simulink model "sistemaMotorCC_PID"  (R2018a)
settings: Solver=FixedStepAuto  StartTime=0.0  StopTime=119.98  RelTol=1e-3
PreLoadFcn:
  | % Motor Parameters
  | 
  | J=0.01;     %kg*m^2
  | b=0.1;      %N*m/(rad/s)
  | K=0.01;     %V/(rad/s)
  | R=1;        %Ohm
  | L=0.5;      %H
libraries: simulink x1
settings Model: Creator=deastman  LastModifiedBy=artur
settings DataIOCC: LimitDataPoints=on  SaveFormat=Array
settings OptimizationCC: ExpressionDepthLimit=2147483647  InitFltsAndDblsToZero=on  LifeSpan=inf
settings DebuggingCC: UnderspecifiedInitializationDetection=Classic  MergeDetectMultiDrivingBlocksExec=none  SolverPrmCheckMsg=warning  FcnCallInpInsideContextMsg=warning  StateNameClashWarn=warning  SFUnexpectedBacktrackingDiag=warning  SFNoUnconditionalDefaultTransitionDiag=warning  SFExecutionAtInitializationDiag=none
settings HardwareCC: ProdBitPerPointer=32  ProdBitPerSizeT=32  ProdBitPerPtrDiffT=32  ProdLargestAtomicFloat=None  ProdIntDivRoundTo=Undefined  ProdEndianess=Unspecified  ProdWordSize=32  ProdHWDeviceType=32-bit Generic
settings ModelReferenceCC: PropagateSignalLabelsOutOfModel=off
settings CodeAppCC: StateflowObjectComments=on
settings GRTTargetCC: TargetLangStandard=C89/C90 (ANSI)  GeneratePreprocessorConditionals=Disable all  CombineOutputUpdateFcns=off  GRTInterface=on
settings ConfigComp: CovMetricSettings=dw  CovHtmlReporting=on  CovSaveCumulativeToWorkspaceVar=on  CovSaveSingleToWorkspaceVar=on  CovExternalEMLEnable=off

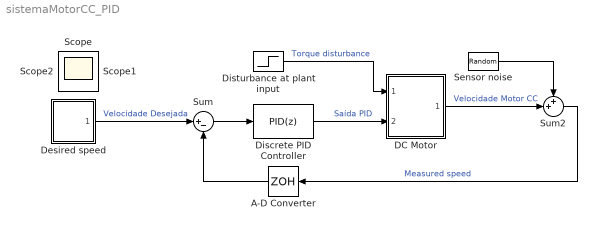
== system sistemaMotorCC_PID ==
  " Disturbance at plant input" : Step  Time=0  After=0  SampleTime=0
  A-D Converter : ZeroOrderHold  SampleTime=0.02
  DC Motor : Subsystem  mask(DC Motor){b=b, J=J, K=K, R=R, L=L}
      mask prompts: b "Damping:"; J "Inertia:"; K "Back EMF:"; R "Resistance:"; L "Inductance:"
      mask help: An ideal model of a DC Motor
      mask Help: This is <b>more elaborate<b> help.
      mask Display: image(imread('dcmotor.jpg'))
  Desired speed : Subsystem
  Discrete PID Controller : simulink/Continuous/PID Controller  Controller=PID  TimeDomain=Discrete-time  SampleTime=0.02  IntegratorMethod=Forward Euler  FilterMethod=Forward Euler  Form=Parallel  UseFilter=on  ControllerParametersSource=internal  P=5.6086  I=17.255  D=0  N=100  InitialConditionSource=internal  InitialConditionForIntegrator=0  InitialConditionForFilter=0  ExternalReset=none  LimitOutput=off  UpperSaturationLimit=10  LowerSaturationLimit=-10  LinearizeAsGain=on  AntiWindupMode=back-calculation  Kb=1  TrackingMode=off  Kt=1  PParamMin=[]  PParamMax=[]  IParamMin=[]  IParamMax=[]  DParamMin=[]  DParamMax=[]  NParamMin=[]  NParamMax=[]  KbParamMin=[]  KbParamMax=[]  KtParamMin=[]  KtParamMax=[]  POutMin=[]  POutMax=[]  IOutMin=[]  IOutMax=[]  DOutMin=[]  DOutMax=[]  NOutMin=[]  NOutMax=[]  KbOutMin=[]  KbOutMax=[]  KtOutMin=[]  KtOutMax=[]  IntegratorOutMin=[]  IntegratorOutMax=[]  FilterOutMin=[]  FilterOutMax=[]  SumOutMin=[]  SumOutMax=[]  SumI1OutMin=[]  SumI1OutMax=[]  SumI2OutMin=[]  SumI2OutMax=[]  SumI3OutMin=[]  SumI3OutMax=[]  SumDOutMin=[]  SumDOutMax=[]  SaturationOutMin=[]  SaturationOutMax=[]  IntegratorContinuousStateAttributes=''  IntegratorStateMustResolveToSignalObject=off  IntegratorRTWStateStorageClass=Auto  FilterContinuousStateAttributes=''  FilterStateMustResolveToSignalObject=off  FilterRTWStateStorageClass=Auto  DifferentiatorICPrevScaledInput=0  DifferentiatorOutMin=[]  DifferentiatorOutMax=[]  FilterDiffOutCoefMin=[]  FilterDiffOutCoefMax=[]  SumDenOutMin=[]  SumDenOutMax=[]  SumNumOutMin=[]  SumNumOutMax=[]  ReciprocalOutMin=[]  ReciprocalOutMax=[]  DivideOutMin=[]  DivideOutMax=[]  TunerSelectOption=Transfer Function Based (PID Tuner App)
  Sensor noise : RandomNumber  Variance=0  SampleTime=0
  Sum : Sum  Inputs=|+-
  Sum2 : Sum  Inputs=++|
  Scope : Scope
  Scope1 : Scope
  Scope2 : Scope
  wires:
  " Disturbance at plant input"/1 -> DC Motor/1(Torque)  "Torque disturbance"
  Sum/1 -> Discrete PID Controller/1
  Discrete PID Controller/1 -> DC Motor/2(Voltage)  "Saída PID"
  Desired speed/1(Speed) -> Sum/1  "Velocidade Desejada"
  DC Motor/1(Speed) -> Sum2/2  "Velocidade Motor CC"
  Sum2/1 -> A-D Converter/1  "Measured speed"
  Sensor noise/1 -> Sum2/1
  A-D Converter/1 -> Sum/2

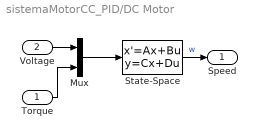
== system sistemaMotorCC_PID/DC Motor ==
  Torque : Inport
  Voltage : Inport  Port=2
  Mux : Mux  Inputs=2
  State-Space : StateSpace  A=[-b/J K/J; -K/L -R/L]  B=[0 -1/J; 1/L 0]  C=[1 0]  D=[0 0]  InitialCondition=0
  Speed : Outport
  wires:
  Mux/1 -> State-Space/1
  Voltage/1 -> Mux/1
  State-Space/1 -> Speed/1  "w"
  Torque/1 -> Mux/2

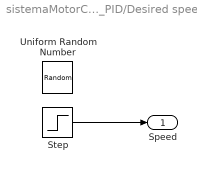
== system sistemaMotorCC_PID/Desired speed ==
  Step : Step  Time=0  SampleTime=0
  Uniform Random Number : UniformRandomNumber  Minimum=-5  Maximum=5  Seed=1  SampleTime=6
  Speed : Outport
  wires:
  Step/1 -> Speed/1
